simulink model "RPL_3D_ModeCompl"  (R2021b)
settings: Solver=VariableStepAuto  StartTime=0.0  StopTime=20  RelTol=1e-3
values from neighbouring files (symbols this model uses):
  Ar = pi*R_rad^2    (= 0.00282743338823)    [constants1DoF.m]
  Cd = 0.5    [constants1DoF.m]
  g = 9.81    [constants1DoF.m]
  m_d_c = 0.01    [constants1DoF.m]
  m_r = 0.5    [constants1DoF.m]
  rho = 1.225    [constants1DoF.m]
  t_burn = 2    [constants1DoF.m]
  Tmax = 10    [constants1DoF.m]
libraries: aerolibanim x1
settings Model: Creator=josepfamador  LastModifiedBy=josepfamador
settings SolverCC: AlgebraicLoopSolver=TrustRegion
settings DebuggingCC: SFMachineParentedDataDiag=warning

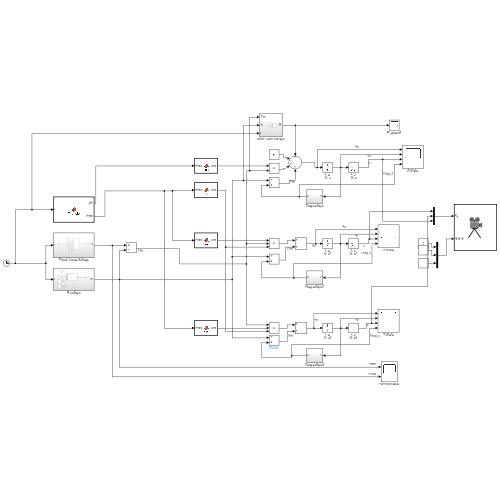
[thumbnail: Simulink's stored preview of the top-level diagram]
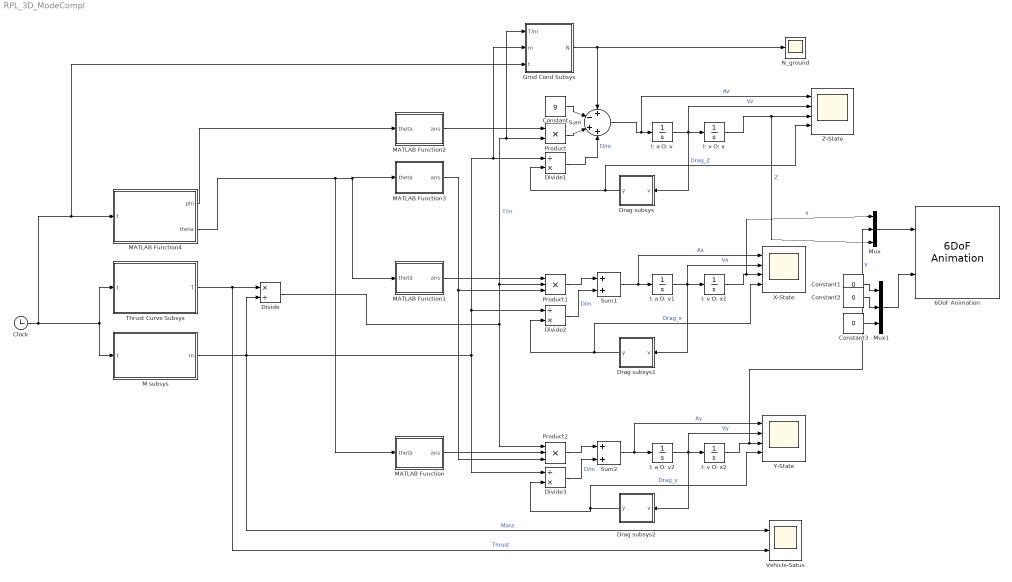
== system RPL_3D_ModeCompl ==
  6DoF Animation : aerolibanim/6DoF Animation  u1=[-400 400 -200 200 -500 -300]  u2=0.1  u3=10  u4=[0 0 0]  u5=Cockpit  u6=[200 200 -250]  u7=10  u8=on
  Clock : Clock
      settings: Decimation=5
  Constant : Constant  Value=g
  Constant1 : Constant  Value=0
  Constant2 : Constant  Value=0
  Constant3 : Constant  Value=0
  Divide : Product  Inputs=*/
  Divide1 : Product  Inputs=/*
  Divide2 : Product  Inputs=/*
  Divide3 : Product  Inputs=/*
  Drag subsys : Subsystem
  Drag subsys1 : Subsystem
  Drag subsys2 : Subsystem
  Grnd Cond Subsys : Subsystem
  I: a O: v : Integrator
  I: a O: v1 : Integrator
  I: a O: v2 : Integrator
  I: v O: x : Integrator  LimitOutput=on  LowerSaturationLimit=0
  I: v O: x1 : Integrator  LimitOutput=on  LowerSaturationLimit=0
  I: v O: x2 : Integrator  LimitOutput=on  LowerSaturationLimit=0
  M subsys : Subsystem
  MATLAB Function : MATLAB Function  TreatAsAtomicUnit=on
  MATLAB Function1 : MATLAB Function  TreatAsAtomicUnit=on
  MATLAB Function2 : MATLAB Function  TreatAsAtomicUnit=on
  MATLAB Function3 : MATLAB Function  TreatAsAtomicUnit=on
  MATLAB Function4 : MATLAB Function  TreatAsAtomicUnit=on
  Mux : Mux  Inputs=3
  Mux1 : Mux  Inputs=3
  N_ground : Scope
  Product : Product
  Product1 : Product  Inputs=3
  Product2 : Product  Inputs=3
  Sum : Sum  Inputs=+-++
  Sum1 : Sum
  Sum2 : Sum
  Thrust Curve Subsys : Subsystem
  Vehicle-Satus : Scope  NumInputPorts=2
  X-State : Scope  NumInputPorts=4
  Y-State : Scope  NumInputPorts=4
  Z-State : Scope  NumInputPorts=4
  wires:
  Clock/1 -> Thrust Curve Subsys/1(t), M subsys/1(t), Grnd Cond Subsys/3(t), MATLAB Function4/1(t)
  Constant/1 -> Sum/2
  Sum/1 -> Z-State/1, I: a O: v/1  "Az"
  I: a O: v/1 -> Drag subsys/1(v), Z-State/2, I: v O: x/1  "Vz"
  Divide/1 -> Product/2, Grnd Cond Subsys/1(T/m), Product1/2, Product2/1  "T/m"
  Divide1/1 -> Sum/4  "D/m"
  M subsys/1(m) -> Vehicle-Satus/1, Grnd Cond Subsys/2(m), Divide1/1, Divide2/1, Divide3/1, Divide/2  "Mass"
  Thrust Curve Subsys/1(T) -> Vehicle-Satus/2, Divide/1  "Thrust"
  Drag subsys/1(y) -> Z-State/4, Divide1/2  "Drag_Z"
  Sum1/1 -> X-State/1, I: a O: v1/1  "Ax"
  Drag subsys1/1(y) -> X-State/4, Divide2/2  "Drag_x"
  Divide2/1 -> Sum1/2  "D/m"
  Sum2/1 -> Y-State/1, I: a O: v2/1  "Ay"
  Drag subsys2/1(y) -> Divide3/2, Y-State/4  "Drag_y"
  I: a O: v2/1 -> Y-State/2, I: v O: x2/1, Drag subsys2/1(v)  "Vy"
  Divide3/1 -> Sum2/2  "D/m"
  MATLAB Function1/1(ans) -> Product1/1
  MATLAB Function/1(ans) -> Product2/2
  Product2/1 -> Sum2/1
  Product1/1 -> Sum1/1
  Product/1 -> Sum/3
  MATLAB Function2/1(ans) -> Product/1
  MATLAB Function3/1(ans) -> Product2/3, Product1/3
  MATLAB Function4/1(phi) -> MATLAB Function2/1(theta)
  MATLAB Function4/2(theta) -> MATLAB Function1/1(theta), MATLAB Function3/1(theta), MATLAB Function/1(theta)
  Grnd Cond Subsys/1(N) -> Sum/1, N_ground/1
  I: a O: v1/1 -> I: v O: x1/1, Drag subsys1/1(v), X-State/2  "Vx"
  I: v O: x2/1 -> Mux/2, Y-State/3  "y"
  I: v O: x/1 -> Mux/3, Z-State/3  "Z"
  I: v O: x1/1 -> Mux/1, X-State/3  "x"
  Mux/1 -> 6DoF Animation/1
  Constant1/1 -> Mux1/1
  Constant2/1 -> Mux1/2
  Constant3/1 -> Mux1/3
  Mux1/1 -> 6DoF Animation/2

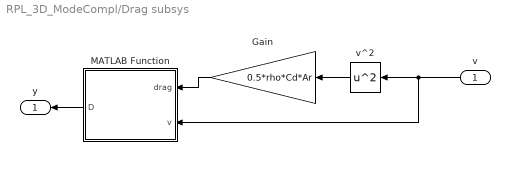
== system RPL_3D_ModeCompl/Drag subsys ==
  v : Inport
  Gain : Gain  Gain=0.5*rho*Cd*Ar
  MATLAB Function : MATLAB Function  TreatAsAtomicUnit=on
  v^2 : Math  Operator=square  SaturateOnIntegerOverflow=on
  y : Outport
  wires:
  v^2/1 -> Gain/1
  v/1 -> MATLAB Function/2(v), v^2/1
  Gain/1 -> MATLAB Function/1(drag)
  MATLAB Function/1(D) -> y/1

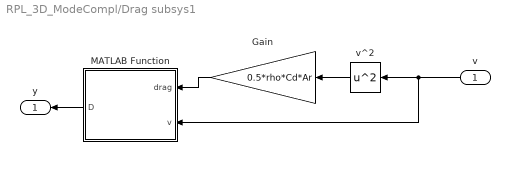
== system RPL_3D_ModeCompl/Drag subsys1 ==
  v : Inport
  Gain : Gain  Gain=0.5*rho*Cd*Ar
  MATLAB Function : MATLAB Function  TreatAsAtomicUnit=on
  v^2 : Math  Operator=square  SaturateOnIntegerOverflow=on
  y : Outport
  wires:
  v^2/1 -> Gain/1
  v/1 -> MATLAB Function/2(v), v^2/1
  Gain/1 -> MATLAB Function/1(drag)
  MATLAB Function/1(D) -> y/1

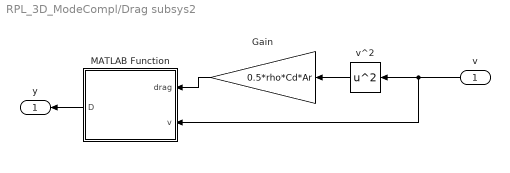
== system RPL_3D_ModeCompl/Drag subsys2 ==
  v : Inport
  Gain : Gain  Gain=0.5*rho*Cd*Ar
  MATLAB Function : MATLAB Function  TreatAsAtomicUnit=on
  v^2 : Math  Operator=square  SaturateOnIntegerOverflow=on
  y : Outport
  wires:
  v^2/1 -> Gain/1
  v/1 -> MATLAB Function/2(v), v^2/1
  Gain/1 -> MATLAB Function/1(drag)
  MATLAB Function/1(D) -> y/1

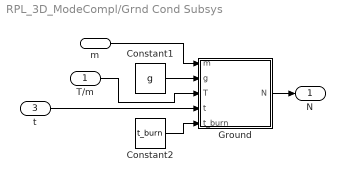
== system RPL_3D_ModeCompl/Grnd Cond Subsys ==
  T/m : Inport
  m : Inport  Port=2
  t : Inport  Port=3
  Constant1 : Constant  Value=g
  Constant2 : Constant  Value=t_burn
  Ground : MATLAB Function  TreatAsAtomicUnit=on
  N : Outport
  wires:
  m/1 -> Ground/1(m)
  Constant2/1 -> Ground/5(t_burn)
  t/1 -> Ground/4(t)
  Ground/1(N) -> N/1
  T/m/1 -> Ground/3(T)
  Constant1/1 -> Ground/2(g)

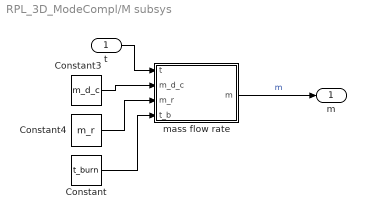
== system RPL_3D_ModeCompl/M subsys ==
  t : Inport
  Constant : Constant  Value=t_burn
  Constant3 : Constant  Value=m_d_c
  Constant4 : Constant  Value=m_r
  mass flow rate : MATLAB Function  TreatAsAtomicUnit=on
  m : Outport
  wires:
  t/1 -> mass flow rate/1(t)
  Constant3/1 -> mass flow rate/2(m_d_c)
  Constant4/1 -> mass flow rate/3(m_r)
  mass flow rate/1(m) -> m/1  "m"
  Constant/1 -> mass flow rate/4(t_b)

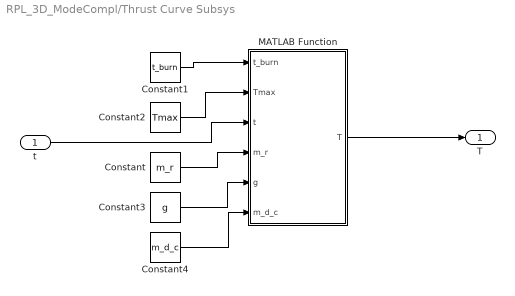
== system RPL_3D_ModeCompl/Thrust Curve Subsys ==
  t : Inport
  Constant : Constant  Value=m_r
  Constant1 : Constant  Value=t_burn
  Constant2 : Constant  Value=Tmax
  Constant3 : Constant  Value=g
  Constant4 : Constant  Value=m_d_c
  MATLAB Function : MATLAB Function  TreatAsAtomicUnit=on
  T : Outport
  wires:
  Constant1/1 -> MATLAB Function/1(t_burn)
  Constant2/1 -> MATLAB Function/2(Tmax)
  t/1 -> MATLAB Function/3(t)
  MATLAB Function/1(T) -> T/1
  Constant/1 -> MATLAB Function/4(m_r)
  Constant3/1 -> MATLAB Function/5(g)
  Constant4/1 -> MATLAB Function/6(m_d_c)

== matlab function RPL_3D_ModeCompl/M subsys/mass flow rate ==
  data: t input; m output; m_d_c input; m_r input; t_b input
function m = m_flow(t, m_d_c, m_r, t_b)
%Const Define in 'constants1DoF.m'
%out mass at time t


if t <= t_b 
    m= -m_d_c*t + m_r;
else
    m = -m_d_c*t_b + m_r;
end

== matlab function RPL_3D_ModeCompl/Thrust Curve Subsys/MATLAB Function ==
  data: t_burn input; Tmax input; t input; T output; m_r input; g input; m_d_c input
function T = T_of_t(t_burn, Tmax, t, m_r, g, m_d_c)
%Approx Thurst Curve.
%Total Burn time = 1s
%Max Thrust 100N

%Constants Defined in 'constants1DoF.m'
x_hf = t_burn/2;
a = Tmax/((x_hf)*(x_hf - t_burn));


if t<=0
    T = 0; %ded

elseif t<t_burn
    T = a*t*(t-t_burn); %lift off burn

else
    T = m_r*g - t_burn*m_d_c; %constant burn at rocket weight
end

== matlab function RPL_3D_ModeCompl/Drag subsys/MATLAB Function ==
  data: drag input; D output; v input
function D = sign_change(drag, v)
%changes signs of Drag when appropiate. Vertical Up is positive
if v>0
    D = -drag;
else
    D = drag;
end

== matlab function RPL_3D_ModeCompl/Drag subsys1/MATLAB Function ==
  data: drag input; D output; v input
function D = sign_change(drag, v)
%changes signs of Drag when appropiate.
if v>0
    D = -drag;
else
    D = drag;
end

== matlab function RPL_3D_ModeCompl/Drag subsys2/MATLAB Function ==
  data: drag input; D output; v input
function D = sign_change(drag, v)
%changes signs of Drag when appropiate. Vertical Up is positive
if v>0
    D = -drag;
else
    D = drag;
end

== matlab function RPL_3D_ModeCompl/MATLAB Function ==
  data: theta input; ans output
function ans = sin(theta)
%in rad
ans = sin(theta);

== matlab function RPL_3D_ModeCompl/MATLAB Function1 ==
  data: theta input; ans output
function ans = cos(theta)
%in rad
ans = cos(theta);

== matlab function RPL_3D_ModeCompl/MATLAB Function2 ==
  data: theta input; ans output
function ans = cos(theta)
%in rad
ans = cos(theta);

== matlab function RPL_3D_ModeCompl/MATLAB Function3 ==
  data: theta input; ans output
function ans = sin(theta)
%in rad
ans = sin(theta);

== matlab function RPL_3D_ModeCompl/MATLAB Function4 ==
  data: t input; phi output; theta output
function [phi,theta] = T_angle(t)

dummyconst = 1; %random debug/test const.

theta = dummyconst * t;
phi = 0.25;

== matlab function RPL_3D_ModeCompl/Grnd Cond Subsys/Ground ==
  data: N output; m input; g input; T input; t input; t_burn input
function N = grnd(m,g,T,t,t_burn)

%ground Normal Force.
W = m*g;

if T < W && t<t_burn/2
    N = g - T/m;
else
    N = 0;
end
